simulink model "AlarmConditionEnable_HatchOpen"  (R2020a)
settings: Solver=VariableStepAuto  StartTime=0.0  StopTime=inf  RelTol=1e-3
settings Model: Creator=99003727  LastModifiedBy=99003727

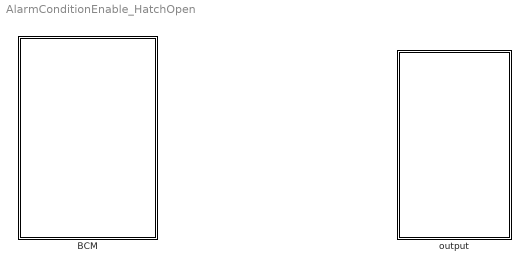
== system AlarmConditionEnable_HatchOpen ==
  BCM : Subsystem
  output : Subsystem

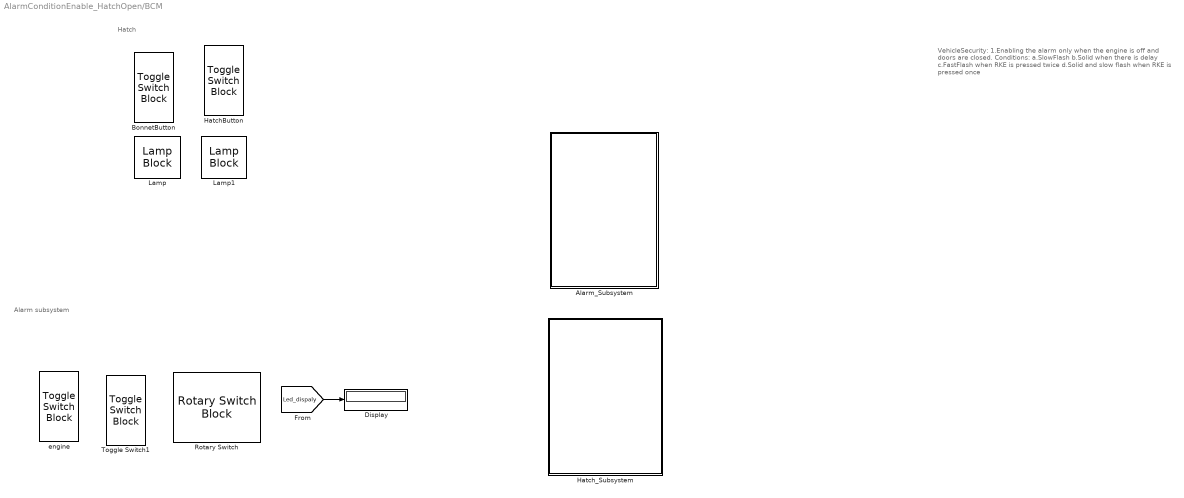
== system AlarmConditionEnable_HatchOpen/BCM ==
  note: VehicleSecurity:
      | 1.Enabling the alarm only when the engine is off
      | and doors are closed.
      | Conditions:
      | a.SlowFlash
      | b.Solid when there is delay
      | c.FastFlash when RKE is pressed twice
      | d.Solid and slow flash when RKE is pressed once
  note: Alarm subsystem
  note: Hatch
  Alarm_Subsystem : Subsystem
  BonnetButton : ToggleSwitchBlock
      settings: Values={{'Off', 'On'}, [0 1]}
  Display : Display
  HatchButton : ToggleSwitchBlock
      settings: Values={{'Off', 'On'}, [0 1]}
  Hatch_Subsystem : Subsystem
  Lamp : LampBlock
  Lamp1 : LampBlock
  Rotary Switch : RotarySwitchBlock
      settings: Values={{'solidOff', 'single press', 'doublePress'}, [0 1 2]}
  Toggle Switch1 : ToggleSwitchBlock
      settings: Values={{'Off', 'On'}, [0 1]}
  engine : ToggleSwitchBlock
      settings: Values={{'Off', 'On'}, [0 1]}
  wires:
  [Led_dispaly] -> Display/1

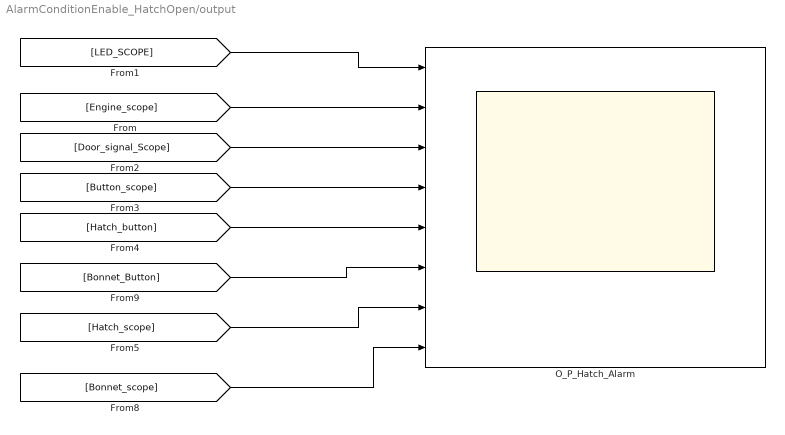
== system AlarmConditionEnable_HatchOpen/output ==
  O_P_Hatch_Alarm : Scope  NumInputPorts=8
  wires:
  [LED_SCOPE] -> O_P_Hatch_Alarm/1
  [Engine_scope] -> O_P_Hatch_Alarm/2
  [Door_signal_Scope] -> O_P_Hatch_Alarm/3
  [Button_scope] -> O_P_Hatch_Alarm/4
  [Hatch_button] -> O_P_Hatch_Alarm/5
  [Bonnet_Button] -> O_P_Hatch_Alarm/6
  [Hatch_scope] -> O_P_Hatch_Alarm/7
  [Bonnet_scope] -> O_P_Hatch_Alarm/8

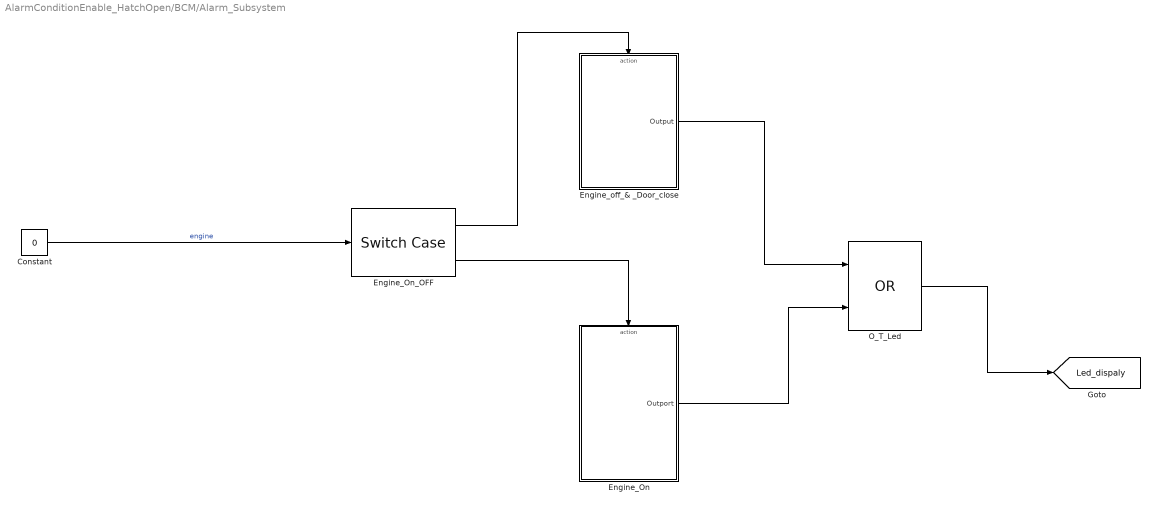
== system AlarmConditionEnable_HatchOpen/BCM/Alarm_Subsystem ==
  Constant : Constant  Value=0
  Engine_On : Subsystem  TreatAsAtomicUnit=on
  Engine_On_OFF : SwitchCase  CaseConditions={0,1}  ShowDefaultCase=off
  Engine_off_& _Door_close : Subsystem  TreatAsAtomicUnit=on
  O_T_Led : Logic  Operator=OR  IconShape=distinctive  AllPortsSameDT=off  OutDataTypeStr=boolean
  tag scope: Led_dispaly=global
  wires:
  O_T_Led/1 -> [Led_dispaly]
  Engine_On_OFF/1 -> Engine_off_& _Door_close/Action
  Engine_On_OFF/2 -> Engine_On/Action
  Engine_On/1(Outport) -> O_T_Led/2
  Engine_off_& _Door_close/1(Output) -> O_T_Led/1
  Constant/1 -> Engine_On_OFF/1  "engine"

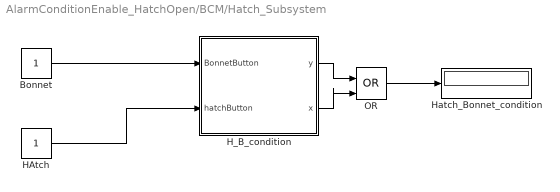
== system AlarmConditionEnable_HatchOpen/BCM/Hatch_Subsystem ==
  Bonnet : Constant
  HAtch : Constant
  H_B_condition : Stateflow chart  TreatAsAtomicUnit=on
  Hatch_Bonnet_condition : Display
  OR : Logic  Operator=OR  IconShape=distinctive  AllPortsSameDT=off  OutDataTypeStr=boolean
  wires:
  Bonnet/1 -> H_B_condition/1(BonnetButton)
  OR/1 -> Hatch_Bonnet_condition/1
  H_B_condition/1(y) -> OR/1
  H_B_condition/2(x) -> OR/2
  HAtch/1 -> H_B_condition/2(hatchButton)

== system AlarmConditionEnable_HatchOpen/BCM/Alarm_Subsystem/Engine_On ==
  Action Port : ActionPort  ActionPortLabel=case [ 1 ]:
  Enigine_Off : Constant  Value=0
  Outport : Outport
  wires:
  Enigine_Off/1 -> Outport/1

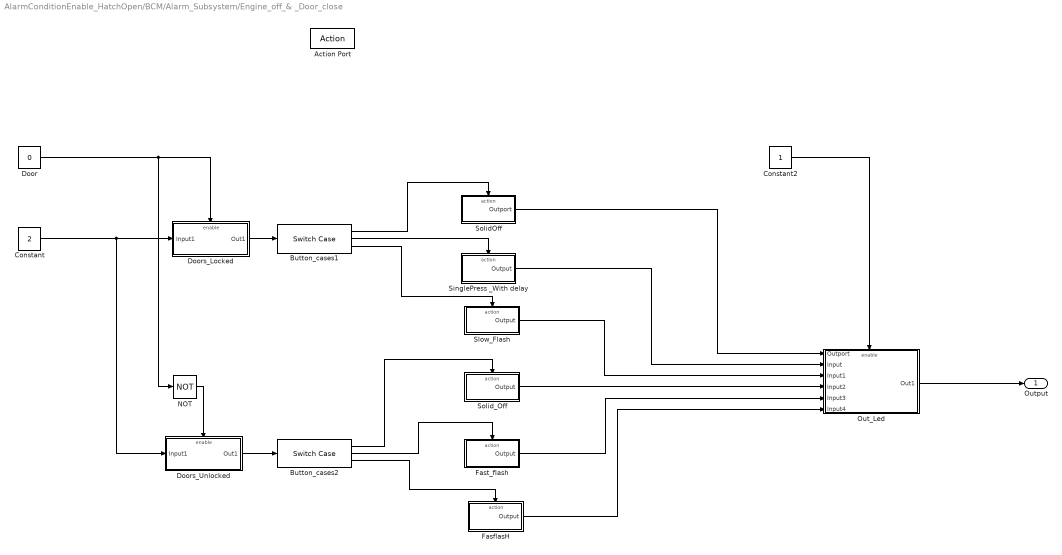
== system AlarmConditionEnable_HatchOpen/BCM/Alarm_Subsystem/Engine_off_& _Door_close ==
  Action Port : ActionPort  ActionPortLabel=case [ 0 ]:
  " SolidOff" : Subsystem  TreatAsAtomicUnit=on
  Button_cases1 : SwitchCase  CaseConditions={0,1,2}  ShowDefaultCase=off
  Button_cases2 : SwitchCase  CaseConditions={0,1,2}  ShowDefaultCase=off
  Constant : Constant  Value=2
  Constant2 : Constant
  Door : Constant  Value=0
  Doors_Locked : Subsystem  TreatAsAtomicUnit=on
  Doors_Unlocked : Subsystem  TreatAsAtomicUnit=on
  FasflasH : Subsystem  TreatAsAtomicUnit=on
  Fast_flash : Subsystem  TreatAsAtomicUnit=on
  NOT : Logic  Operator=NOT  IconShape=distinctive  AllPortsSameDT=off  OutDataTypeStr=boolean
  Out_Led : Subsystem  TreatAsAtomicUnit=on
  SinglePress _With delay : Subsystem  TreatAsAtomicUnit=on
  Slow_Flash : Subsystem  TreatAsAtomicUnit=on
  Solid_Off : Subsystem  TreatAsAtomicUnit=on
  Output : Outport
  wires:
  Out_Led/1(Out1) -> Output/1
  Button_cases1/1 -> " SolidOff"/Action
  Button_cases1/2 -> SinglePress _With delay/Action
  Button_cases1/3 -> Slow_Flash/Action
  Doors_Locked/1(Out1) -> Button_cases1/1
  NOT/1 -> Doors_Unlocked/Enable
  Doors_Unlocked/1(Out1) -> Button_cases2/1
  Button_cases2/1 -> Solid_Off/Action
  Button_cases2/2 -> Fast_flash/Action
  Button_cases2/3 -> FasflasH/Action
  Constant2/1 -> Out_Led/Enable
  Slow_Flash/1(Output) -> Out_Led/3(Input1)
  Fast_flash/1(Output) -> Out_Led/5(Input3)
  FasflasH/1(Output) -> Out_Led/6(Input4)
  SinglePress _With delay/1(Output) -> Out_Led/2(Input)
  Solid_Off/1(Output) -> Out_Led/4(Input2)
  " SolidOff"/1(Outport) -> Out_Led/1(Outport)
  Door/1 -> NOT/1, Doors_Locked/Enable
  Constant/1 -> Doors_Unlocked/1(Input1), Doors_Locked/1(Input1)

== system AlarmConditionEnable_HatchOpen/BCM/Alarm_Subsystem/Engine_off_& _Door_close/ SolidOff ==
  Action Port : ActionPort  ActionPortLabel=case [ 0 ]:
  Constant : Constant  Value=0
  Outport : Outport
  wires:
  Constant/1 -> Outport/1

== system AlarmConditionEnable_HatchOpen/BCM/Alarm_Subsystem/Engine_off_& _Door_close/Doors_Locked ==
  Input1 : Inport
  Enable : EnablePort
  Out1 : Outport
  wires:
  Input1/1 -> Out1/1

== system AlarmConditionEnable_HatchOpen/BCM/Alarm_Subsystem/Engine_off_& _Door_close/Doors_Unlocked ==
  Input1 : Inport
  Enable : EnablePort
  Out1 : Outport
  wires:
  Input1/1 -> Out1/1

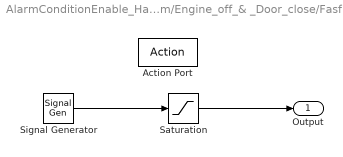
== system AlarmConditionEnable_HatchOpen/BCM/Alarm_Subsystem/Engine_off_& _Door_close/FasflasH ==
  Action Port : ActionPort  ActionPortLabel=case [ 2 ]:
  Saturation : Saturate  UpperLimit=1  LowerLimit=0
  Signal Generator : SignalGenerator
  Output : Outport
  wires:
  Saturation/1 -> Output/1
  Signal Generator/1 -> Saturation/1

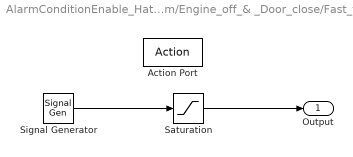
== system AlarmConditionEnable_HatchOpen/BCM/Alarm_Subsystem/Engine_off_& _Door_close/Fast_flash ==
  Action Port : ActionPort  ActionPortLabel=case [ 1 ]:
  Saturation : Saturate  UpperLimit=1  LowerLimit=0
  Signal Generator : SignalGenerator  WaveForm=square
  Output : Outport
  wires:
  Saturation/1 -> Output/1
  Signal Generator/1 -> Saturation/1

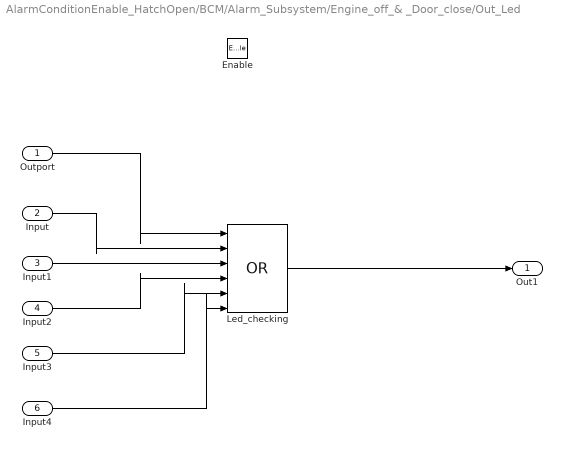
== system AlarmConditionEnable_HatchOpen/BCM/Alarm_Subsystem/Engine_off_& _Door_close/Out_Led ==
  Outport : Inport
  Input : Inport  Port=2
  Input1 : Inport  Port=3
  Input2 : Inport  Port=4
  Input3 : Inport  Port=5
  Input4 : Inport  Port=6
  Enable : EnablePort
  Led_checking : Logic  Operator=OR  Inputs=6  IconShape=distinctive  AllPortsSameDT=off  OutDataTypeStr=boolean
  Out1 : Outport
  wires:
  Outport/1 -> Led_checking/1
  Input/1 -> Led_checking/2
  Input1/1 -> Led_checking/3
  Input2/1 -> Led_checking/4
  Input3/1 -> Led_checking/5
  Input4/1 -> Led_checking/6
  Led_checking/1 -> Out1/1

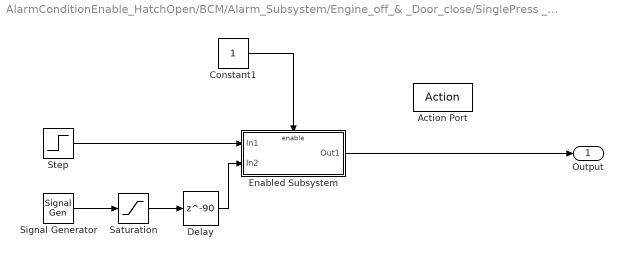
== system AlarmConditionEnable_HatchOpen/BCM/Alarm_Subsystem/Engine_off_& _Door_close/SinglePress _With delay ==
  Action Port : ActionPort  ActionPortLabel=case [ 1 ]:
  Constant1 : Constant
  Delay : Delay  DelayLength=90
  Enabled Subsystem : Subsystem  TreatAsAtomicUnit=on
  Saturation : Saturate  UpperLimit=1  LowerLimit=0
  Signal Generator : SignalGenerator  WaveForm=square  Frequency=0.5
  Step : Step  Time=30  Before=1  After=0  SampleTime=0
  Output : Outport
  wires:
  Enabled Subsystem/1(Out1) -> Output/1
  Delay/1 -> Enabled Subsystem/2(In2)
  Saturation/1 -> Delay/1
  Constant1/1 -> Enabled Subsystem/Enable
  Signal Generator/1 -> Saturation/1
  Step/1 -> Enabled Subsystem/1(In1)

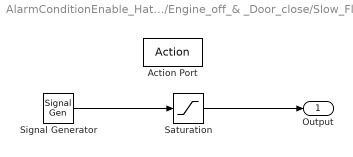
== system AlarmConditionEnable_HatchOpen/BCM/Alarm_Subsystem/Engine_off_& _Door_close/Slow_Flash ==
  Action Port : ActionPort  ActionPortLabel=case [ 2 ]:
  Saturation : Saturate  UpperLimit=1  LowerLimit=0
  Signal Generator : SignalGenerator  WaveForm=square  Frequency=0.5
  Output : Outport
  wires:
  Saturation/1 -> Output/1
  Signal Generator/1 -> Saturation/1

== system AlarmConditionEnable_HatchOpen/BCM/Alarm_Subsystem/Engine_off_& _Door_close/Solid_Off ==
  Action Port : ActionPort  ActionPortLabel=case [ 0 ]:
  Constant : Constant  Value=0
  Output : Outport
  wires:
  Constant/1 -> Output/1

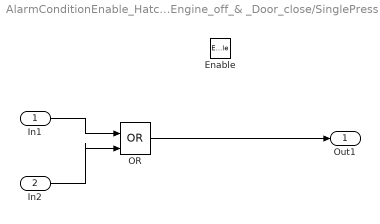
== system AlarmConditionEnable_HatchOpen/BCM/Alarm_Subsystem/Engine_off_& _Door_close/SinglePress _With delay/Enabled Subsystem ==
  In1 : Inport
  In2 : Inport  Port=2
  Enable : EnablePort
  OR : Logic  Operator=OR  IconShape=distinctive  AllPortsSameDT=off  OutDataTypeStr=boolean
  Out1 : Outport
  wires:
  In1/1 -> OR/1
  In2/1 -> OR/2
  OR/1 -> Out1/1

== stateflow chart AlarmConditionEnable_HatchOpen/BCM/Hatch_Subsystem/H_B_condition ==
  state Hatch
    entry:
    if hatchButton==1
    y=1;
    end
    if BonnetButton==1
    x=1;
    end
  state Hatch_off
    entry:
    if hatchButton==0
    y=0;
    end
    if BonnetButton==0
    x=0;
    end
  (default) -> Hatch
  Hatch -> Hatch_off : [BonnetButton==0||hatchButton==0]
  Hatch_off -> Hatch : [BonnetButton==1||hatchButton==1]
  data: BonnetButton input; hatchButton input; y output; x output
